simulink model "Model"  (R2024b)
settings: Solver=ode45  StartTime=0.0  StopTime=90  MaxStep=0.001  RelTol=1e-3
InitFcn:
  | Design
StopFcn:
  | Estimation
undefined symbols (not defined in the file or in its folder): daq, degs2rpm, gbox, Kd, Ki, Kp, LP, mot, RD, rpm2degs, rpm2rads, sens, Tl
libraries: simulink_extras x1
settings Model: Creator=Banaan  LastModifiedBy=Banaan

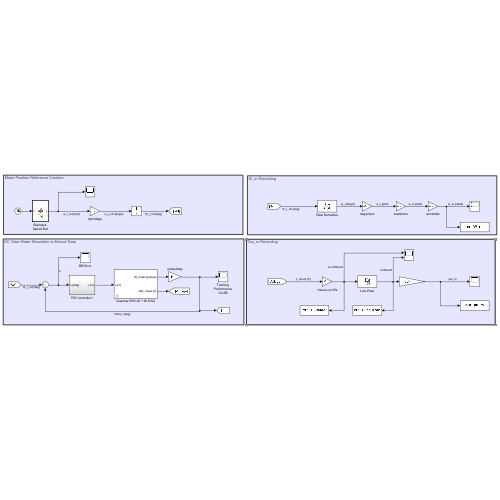
[thumbnail: Simulink's stored preview of the top-level diagram]
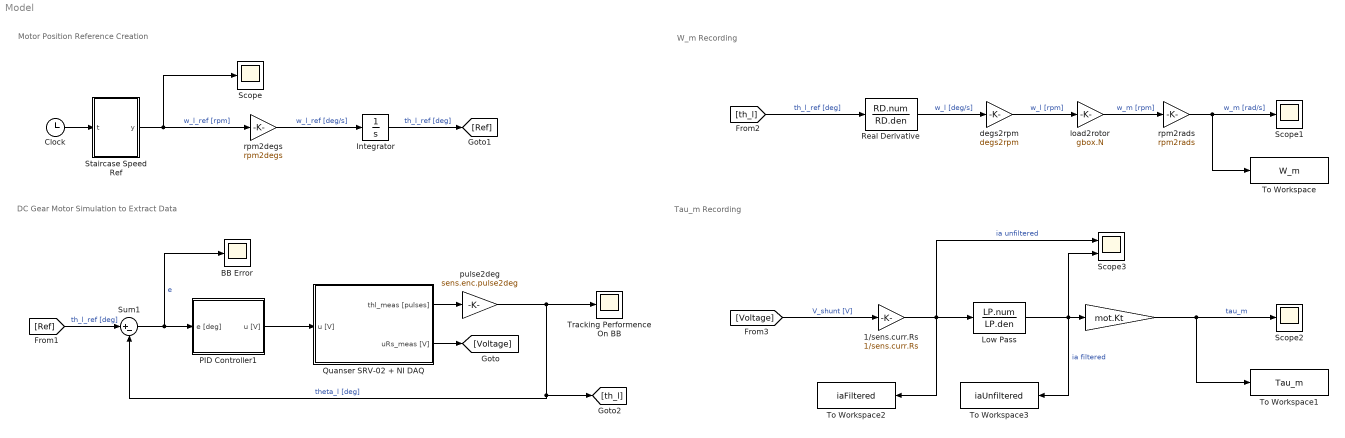
== system Model ==
  note: Tau_m Recording
  note: W_m Recording
  note: DC Gear Motor Simulation to Extract Data
  note: Motor Position Reference Creation
  " " : Gain  Gain=mot.Kt
  1/sens.curr.Rs : Gain  Gain=1/sens.curr.Rs
  BB Error : Scope
  Clock : Clock
  Integrator : Integrator
  Low Pass : TransferFcn  Numerator=LP.num  Denominator=LP.den
  PID Controller1 : Subsystem
  Quanser SRV-02 + NI DAQ : Subsystem  mask(Quanser SRV-02 (with inertial load) + NI DAQ){Ts=0.001, fricType=Coulomb + viscous}
      mask prompts: Ts "NI DAQ Sample Time:"; fricType "Friction model"
      mask help: Quanser SRV-02 (with inertial load) + NI DAQ model.
      mask init:
      | %%  Sensors data
      | 
      | %   shunt resistor
      | sens.curr.Rs = 0.5;                         %   resistance [Ohm]   
      | sens.curr.uRs_std = 0.01;                   %   voltage noise standard dev [V]                           
      | sens.curr.uRs_var = sens.curr.uRs_std^2;	%   voltage noise variance [V^2]
      | 
      | %   Hewlett-Packard HEDS-5540#A06 optical encoder
      | sens.enc.ppr = 500*4;                       %   pulses per rotation
      | sens.enc.pulse2deg = 360/sens.enc.ppr;      %   [pulses] -> [deg]
      | sens.enc.pulse2rad = 2*pi/sens.enc.ppr;     %   [pulses] -> [rad]
      | sens.enc.deg2pulse = sens.enc.ppr/360;      %   [deg] -> [pulses]
      | sens.enc.rad2pulse = sens.enc.ppr/2/pi;     %   [rad] -> [pulses]
      | 
      | 
      | %%  Data acquisition board (daq) data
      | 
      | %   NI PCI-6221 DAC data
      | daq.dac.bits = 16;                                  %   resolution (bits)
      | daq.dac.fs   = 10;                                  %   full scale 
      | daq.dac.q    = 2*daq.dac.fs/(2^daq.dac.bits-1);     %	quantization
      | 
      | %   NI PCI-6221 ADC data
      | daq.adc.bits = 16;                                  %   resolution (bits)
      | daq.adc.fs   = 10;                                  %   full scale (as set in SLDRT Analog Input block)
      | daq.adc.q    = 2*daq.adc.fs/(2^daq.adc.bits-1);     %   quantization
      mask Help:
      | Riccardo Antonello (antonello@dei.unipd.it)
      | 
      | April 24, 2020
      | 
      | Dept. of Information Engineering, University of Padova
      mask TypeOptions fricType: Coulomb + viscous | Karnopp
  Real Derivative : TransferFcn  Numerator=RD.num  Denominator=RD.den
  Scope : Scope
  Scope1 : Scope
  Scope2 : Scope
  Scope3 : Scope  NumInputPorts=2
  Staircase Speed Ref : MATLAB Function  TreatAsAtomicUnit=on
  Sum1 : Sum  Inputs=|+-
  To Workspace : ToWorkspace  VariableName=W_m  SaveFormat=Timeseries  SampleTime=-1
  To Workspace1 : ToWorkspace  VariableName=Tau_m  SaveFormat=Timeseries  SampleTime=-1
  To Workspace2 : ToWorkspace  VariableName=iaFiltered  SaveFormat=Timeseries  SampleTime=-1
  To Workspace3 : ToWorkspace  VariableName=iaUnfiltered  SaveFormat=Timeseries  SampleTime=-1
  Tracking Performence On BB : Scope
  degs2rpm : Gain  Gain=degs2rpm
  load2rotor : Gain  Gain=gbox.N
  pulse2deg : Gain  Gain=sens.enc.pulse2deg
  rpm2degs : Gain  Gain=rpm2degs
  rpm2rads : Gain  Gain=rpm2rads
  wires:
  Quanser SRV-02 + NI DAQ/1(thl_meas [pulses]) -> pulse2deg/1
  pulse2deg/1 -> Tracking Performence On BB/1, Sum1/2, [th_l]  "theta_l [deg]"
  Quanser SRV-02 + NI DAQ/2(uRs_meas [V]) -> [Voltage]
  Sum1/1 -> BB Error/1, PID Controller1/1(e [deg])  "e"
  PID Controller1/1(u [V]) -> Quanser SRV-02 + NI DAQ/1(u [V])
  [Ref] -> Sum1/1  "th_l_ref [deg]"
  Clock/1 -> Staircase Speed Ref/1(t)
  Staircase Speed Ref/1(y) -> Scope/1, rpm2degs/1  "w_l_ref [rpm]"
  rpm2degs/1 -> Integrator/1  "w_l_ref [deg/s]"
  Integrator/1 -> [Ref]  "th_l_ref [deg]"
  Real Derivative/1 -> degs2rpm/1  "w_l [deg/s]"
  degs2rpm/1 -> load2rotor/1  "w_l [rpm]"
  load2rotor/1 -> rpm2rads/1  "w_m [rpm]"
  rpm2rads/1 -> To Workspace/1, Scope1/1  "w_m [rad/s]"
  [th_l] -> Real Derivative/1  "th_l_ref [deg]"
  [Voltage] -> 1/sens.curr.Rs/1  "V_shunt [V]"
  " "/1 -> Scope2/1, To Workspace1/1  "tau_m"
  Low Pass/1 -> To Workspace3/1, Scope3/2, " "/1  "ia filtered"
  1/sens.curr.Rs/1 -> To Workspace2/1, Scope3/1, Low Pass/1  "ia unfiltered"

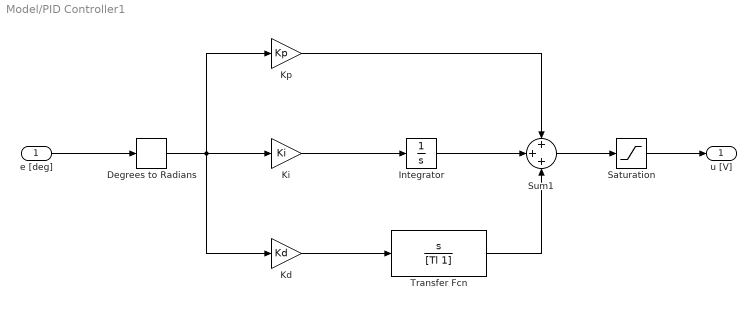
== system Model/PID Controller1 ==
  e [deg] : Inport
  Degrees to Radians : simulink_extras/Transformations/Degrees to Radians
  Integrator : Integrator
  Kd : Gain  Gain=Kd
  Ki : Gain  Gain=Ki
  Kp : Gain  Gain=Kp
  Saturation : Saturate  UpperLimit=daq.adc.fs  LowerLimit=-daq.adc.fs
  Sum1 : Sum  Inputs=+++
  Transfer Fcn : TransferFcn  Numerator=[1 0]  Denominator=[Tl 1]
  u [V] : Outport
  wires:
  Degrees to Radians/1 -> Kd/1, Ki/1, Kp/1
  Transfer Fcn/1 -> Sum1/3
  Integrator/1 -> Sum1/2
  Kd/1 -> Transfer Fcn/1
  Ki/1 -> Integrator/1
  Kp/1 -> Sum1/1
  Sum1/1 -> Saturation/1
  e [deg]/1 -> Degrees to Radians/1
  Saturation/1 -> u [V]/1

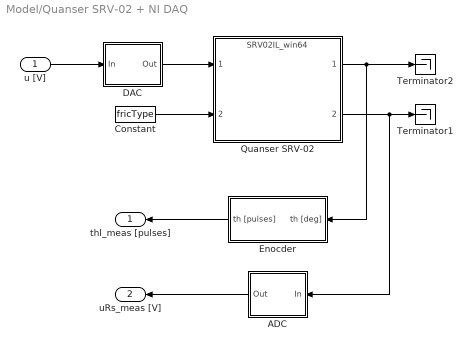
== system Model/Quanser SRV-02 + NI DAQ ==
  u [V] : Inport
  ADC : Subsystem
  Constant : Constant  Value=fricType
  DAC : Subsystem
  Enocder : Subsystem
  Quanser SRV-02 : ModelReference  ModelNameDialog=SRV02IL_win64.slxp  ModelReferenceVersion=1.44  CopyOfModelProtected=on
  Terminator1 : Terminator
  Terminator2 : Terminator
  thl_meas [pulses] : Outport
  uRs_meas [V] : Outport  Port=2
  wires:
  Enocder/1(th [pulses]) -> thl_meas [pulses]/1
  ADC/1(Out) -> uRs_meas [V]/1
  DAC/1(Out) -> Quanser SRV-02/1
  Quanser SRV-02/2 -> ADC/1(In), Terminator1/1
  u [V]/1 -> DAC/1(In)
  Quanser SRV-02/1 -> Enocder/1(th [deg]), Terminator2/1
  Constant/1 -> Quanser SRV-02/2

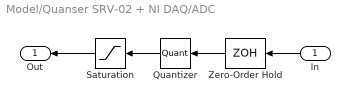
== system Model/Quanser SRV-02 + NI DAQ/ADC ==
  In : Inport
  Quantizer : Quantizer  QuantizationInterval=daq.adc.q
  Saturation : Saturate  UpperLimit=daq.adc.fs  LowerLimit=-daq.adc.fs
  Zero-Order Hold : ZeroOrderHold  SampleTime=Ts
  Out : Outport
  wires:
  Saturation/1 -> Out/1
  In/1 -> Zero-Order Hold/1
  Quantizer/1 -> Saturation/1
  Zero-Order Hold/1 -> Quantizer/1

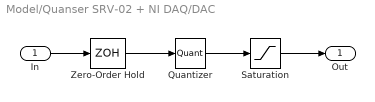
== system Model/Quanser SRV-02 + NI DAQ/DAC ==
  In : Inport
  Quantizer : Quantizer  QuantizationInterval=daq.dac.q
  Saturation : Saturate  UpperLimit=daq.dac.fs  LowerLimit=-daq.dac.fs
  Zero-Order Hold : ZeroOrderHold  SampleTime=Ts
  Out : Outport
  wires:
  Quantizer/1 -> Saturation/1
  In/1 -> Zero-Order Hold/1
  Zero-Order Hold/1 -> Quantizer/1
  Saturation/1 -> Out/1

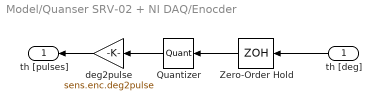
== system Model/Quanser SRV-02 + NI DAQ/Enocder ==
  th [deg] : Inport
  Quantizer : Quantizer  QuantizationInterval=sens.enc.pulse2deg
  Zero-Order Hold : ZeroOrderHold  SampleTime=Ts
  deg2pulse : Gain  Gain=sens.enc.deg2pulse
  th [pulses] : Outport
  wires:
  Quantizer/1 -> deg2pulse/1
  th [deg]/1 -> Zero-Order Hold/1
  Zero-Order Hold/1 -> Quantizer/1
  deg2pulse/1 -> th [pulses]/1

== matlab function Model/Staircase Speed Ref ==
  data: t input; y output
function y = Traj(t)
    if t > 45
        Delta = -50;
        K = ceil(t / 5) - 9;
        y = K * Delta;
    else
        Delta = 50;
        K = ceil(t / 5);
        y = K * Delta;
    end
end
